simulink model "Expriment_Emotion"  (R2014a)
settings: Solver=FixedStepDiscrete  SolverMode=SingleTasking  StartTime=0.0  StopTime=inf  FixedStep=0.01  RelTol=1e-3
PostLoadFcn:
  | h_RPStest = RPStest;
model workspace (MAT data in the model file):
  gtest = 0
undefined symbols (not defined in the file or in its folder): avert, avert_freq_factor, avert_gaze_dirs_chance, avert_gaze_duration_factor, avert_head_frequency_factor, avert_head_speed, BML, BML1, BML2, bmlsL, bmlsM, bodyBusyFlag, clock, emotion_amount_factor, faceBusyFlag, fileID, GAZE_WIN, gazing, mut_freq_factor, mutual_gaze_duration_factor, P, pose_cat_chance, pose_chanc_factor, pose_chance_factor, pose_frequency_factor, pose_lean, pose_lean_flag, pose_space, pose_speed, pose_twitch, pr, serial, STATE_BEFORE, STATE_GO, STATE_OVER, STATE_READY, Stateflow
libraries: simulink x24, instrumentlib x6, realtime_pacer_lib x2, lib_affectiveChar_behavior x1, lib_affectiveChar_input x1
(part 5 of 6)

== stateflow chart Expriment_Emotion/CharacterControl/personalSpace_Controller ==
  state stateInit
    entry: gameState=14;
    TOO_CLOSE=1;TOO_FAR=2;NEUTRAL=0;
    farBuffer=0;closeBuffer=0;neutralBuffer=0;position=1;
    n=encStr2Arr(' ');bmlsM=[n n n n n];newBmlsM=[n n n n n];
    bmlsL=[n n n n n];newBmlsL=[n n n n n];
  note: Problem:
      | Sometimes locomotion BML is sent (visible in the vhmsgYarpRelais) but it is not running. Also smartbody shows duplicate msg id error. It seems that when too many BMLs are sent to smartbody some of them have same IDs.
  state wait
  note: if avert not 1
  state gazeSurprized
    entry: [P,BMLM]=walkInvadingTable(5) ;
    closeBuffer=closeBuffer+1;
    newBmlsM=insertQueue(bmlsM,BMLM);
    bmlsM=newBmlsM;
  state doIt3Times
    entry: position=2;
    closeBuffer=0;
  note: User is too close!
  state headNeuralGazeCamera
    entry: [P,BMLM]=walkInvadingTable(4) ;
    newBmlsM=insertQueue(bmlsM,BMLM);
    bmlsM=newBmlsM;
  state stateWalkBack
    entry:  [P,BMLM]=walkInvadingTable(2);
    newBmlsM=insertQueue(bmlsM,BMLM);  bmlsM=newBmlsM;
    closeBuffer=closeBuffer+1;
  state browUp
    entry: [P,BMLM]=walkInvadingTable(8) ;
    neutralBuffer=neutralBuffer+1;
    newBmlsM=insertQueue(bmlsM,BMLM);
    bmlsM=newBmlsM;
  state doIt3Times1
    entry: position=1;
    neutralBuffer=0;
  note: EXE ORDER IMPORTANT
  state checkUserCoord
  note: correct: [zChange==1]{position=0;}
  state idle
    entry: [P,BMLM]=walkInvadingTable(1);
    newBmlsM=insertQueue(bmlsM,BMLM);
    bmlsM=newBmlsM;
    neutralBuffer=neutralBuffer+1;
  note: User is in the middle!
  state wait2
  state leanFW
    entry: [P,BMLM]=walkInvadingTable(6) ;
    farBuffer=farBuffer+1;
    newBmlsM=insertQueue(bmlsM,BMLM);
    bmlsM=newBmlsM;
  state doIt3Times2
    entry: position=3;
    farBuffer=0;
  note: Problem:
      | We dont know where smatbody is standing (z pos). If smartbody does not run the locomotion BML sent for any reason (too many BMLs), we want to send locomodation BML again after a while to make sure the personal space is correct. On the other hand, we dont want the module to keep sending move bmls.
  state walkFW
    entry:  [P,BMLM]=walkInvadingTable(3) ;
    newBmlsM=insertQueue(bmlsM,BMLM);  bmlsM=newBmlsM;
    farBuffer=farBuffer+1;
  note: User is too far!
  state leanNeutral
    entry:  [P,BMLM]=walkInvadingTable(7) ;
    newBmlsM=insertQueue(bmlsM,BMLM); bmlsM=newBmlsM;
  (default) -> stateInit
  stateInit -> (junction 2)
  wait -> (junction 2)
  (junction 2) -> headNeuralGazeCamera [order 1] : [avert==1]
  (junction 2) -> checkUserCoord [order 2]
  idle -> wait [order 2] : after(5,secs)
  walkFW -> wait [order 2] : after(5,secs)
  stateWalkBack -> wait [order 2] : after(5,secs)
  doIt3Times1 -> wait : after(5,secs)
  doIt3Times2 -> wait : after(5,secs)
  doIt3Times -> wait : after(5,secs)
  checkUserCoord -> (junction 89) [order 3] : [[distance==TOO_CLOSE]&[position~=2]]
  (junction 89) -> gazeSurprized [order 2] : [closeBuffer<2]
  (junction 89) -> stateWalkBack [order 1] : [closeBuffer>=2]
  stateWalkBack -> doIt3Times [order 1] : [closeBuffer==5]
  gazeSurprized -> checkUserCoord
  headNeuralGazeCamera -> checkUserCoord
  checkUserCoord -> (junction 92) [order 2] : [[distance==NEUTRAL]&[position~=1]]
  (junction 92) -> browUp [order 1] : [neutralBuffer<2]
  wait2 -> checkUserCoord [order 1] : [zChange==1]{position=0;}
  idle -> doIt3Times1 [order 1] : [neutralBuffer==5]
  browUp -> checkUserCoord
  (junction 92) -> idle [order 2] : [neutralBuffer>=2]
  wait2 -> checkUserCoord [order 2] : [zChange~=1]
  checkUserCoord -> wait2 [order 4] : after(20,secs)
  checkUserCoord -> (junction 87) [order 1] : [[distance==TOO_FAR]&[position~=3]]
  leanFW -> checkUserCoord
  (junction 87) -> leanFW [order 2] : [farBuffer<2]
  walkFW -> doIt3Times2 [order 1] : [farBuffer==5]
  (junction 87) -> leanNeutral [order 1] : [farBuffer>=2]
  leanNeutral -> walkFW : after(2,secs)
  data: bmls function_input double size=[1000,5]; myBML function_input double size=[1000,1]; newBmls function_output double size=[1000,5]; p function_output double size=1; bmlID function_input double size=1; poseBML function_output double size=[1000,1]; bmls function_input double size=[1000,5]; myBML function_input double size=[1000,1]; newBmls function_output double size=[1000,5]; gameState output double size=1; STATE_READY data_store_memory size=1; STATE_OVER data_store_memory size=1; distance input double size=1; STATE_BEFORE data_store_memory size=1; BML1 data_store_memory size=[256,1]; P data_store_memory; pr data_store_memory; fileID data_store_memory; neutralBuffer local; closeBuffer local; NEUTRAL local; TOO_FAR local; TOO_CLOSE local; farBuffer local; zChange input; position local; avert data_store_memory; newBmlsM local double size=[1000,5]; bmlsM data_store_memory; BMLM local double size=[1000,1]; BMLL local double size=[1000,1]; newBmlsL local double size=[1000,5]; bmlsL data_store_memory; n local
  events: secs input RISING_EDGE_EVENT
  function newBmls =insertQueueLow(bmls,myBML):
    | function newBmls =insertQueueLow(bmls,myBML)
    |     full=1;
    |     t=encStr2Arr(' ');
    |     newBmls=[t t t t t];
    |     for i = 1:5
    |         if (isequal(bmls(:,i),t))
    |             %add to end of the queue where its empty
    |             bmls(:,i)=myBML;
    |             full=0;
    |             break
    |         end
    |     end
    |     if(full~=0)
    |             %if queue full, shift all elements to left which removes the first one, then add to end
    |             bmls(:,1)= bmls(:,2);
    |             bmls(:,2)= bmls(:,3);
    |             bmls(:,3)= bmls(:,4);
    |             bmls(:,5)=myBML;
    |     end
    |     newBmls=bmls;
  function [p,poseBML]=walkInvadingTable(bmlID):
    | function [p,poseBML]=walkInvadingTable(bmlID)
    | 
    | aVarTruthTableCondition_1 = false;
    | aVarTruthTableCondition_2 = false;
    | aVarTruthTableCondition_3 = false;
    | aVarTruthTableCondition_4 = false;
    | aVarTruthTableCondition_5 = false;
    | aVarTruthTableCondition_6 = false;
    | aVarTruthTableCondition_7 = false;
    | aVarTruthTableCondition_8 = false;
    | 
    | 
    | % n
    | 
    | aVarTruthTableCondition_1 = logical(bmlID==1);
    | 
    | % b
    | 
    | aVarTruthTableCondition_2 = logical(bmlID==2);
    | 
    | % f
    | 
    | aVarTruthTableCondition_3 = logical(bmlID==3);
    | 
    | % HN
    | 
    | aVarTruthTableCondition_4 = logical(bmlID==4);
    | 
    | % surprizeGaze
    | 
    | aVarTruthTableCondition_5 = logical(bmlID==5);
    | 
    | % leanFw
    | 
    | aVarTruthTableCondition_6 = logical(bmlID==6);
    | 
    | % leanNeutral
    | 
    | aVarTruthTableCondition_7 = logical(bmlID==7);
    | 
    | % browUp
    | 
    | aVarTruthTableCondition_8 = logical(bmlID==8);
    | 
    | if (aVarTruthTableCondition_1)
    |     aFcnTruthTableAction_1();
    | elseif (aVarTruthTableCondition_2)
    |     aFcnTruthTableAction_2();
    | elseif (aVarTruthTableCondition_3)
    |     aFcnTruthTableAction_3();
    | elseif (aVarTruthTableCondition_4)
    |     aFcnTruthTableAction_4();
    | elseif (aVarTruthTableCondition_5)
    |     aFcnTruthTableAction_5();
    | elseif (aVarTruthTableCondition_6)
    |     aFcnTruthTableAction_6();
    | elseif (aVarTruthTableCondition_7)
    |     aFcnTruthTableAction_7();
    | elseif (aVarTruthTableCondition_8)
    |     aFcnTruthTableAction_8();
    | else % Default
    |     aFcnTruthTableAction_1();
    | end
    | 
    | function aFcnTruthTableAction_1()
    | 
    | % Neutral
    | 
    | poseBML=encStr2Arr( '<?xml version="1.0" ?><act><bml><locomotion manner="walk" facing="gazeTarget"  sbm:accel="0.5" sbm:scootaccel="50" target="0 0"/></bml></act>');p=1;
    | 
    | function aFcnTruthTableAction_2()
    | 
    | % Back
    | 
    | poseBML=encStr2Arr( '<?xml version="1.0" ?><act><bml><locomotion manner="walk"  sbm:accel="0.5" sbm:scootaccel="50" facing="gazeTarget" target="0 -0.6"/></bml></act>');p=1;
    | 
    | function aFcnTruthTableAction_3()
    | 
    | % Forward
    | 
    | poseBML=encStr2Arr( '<?xml version="1.0" ?><act><bml><locomotion manner="walk" facing="gazeTarget"  sbm:accel="0.5" sbm:scootaccel="50" target="0 0.6"/></bml></act>');p=1;
    | 
    | function aFcnTruthTableAction_4()
    | 
    | % NeutralHead
    | 
    | poseBML=encStr2Arr('<?xml version="1.0" ?><act><bml><gaze target="gazeTarget" sbm:joint-range="EYES NECK" sbm:time-hint="1.5"/></bml></act>');p=1;
    | 
    | function aFcnTruthTableAction_5()
    | 
    | % surprisedGaze
    | 
    | poseBML=encStr2Arr('<?xml version="1.0" ?><act><bml><face type="FACS" start="0" end="5" side="BOTH" au="5" relax="3" amount="0.5"/><face type="FACS" start="0" end="5" side="BOTH" au="2" relax="3" amount="0.5"/></bml></act>');p=1;
    | 
    | function aFcnTruthTableAction_6()
    | 
    | % leanFW
    | 
    | poseBML=encStr2Arr('<?xml version="1.0" ?><act><bml><gaze angle="5" direction="DOWN" sbm:joint-range="HEAD BACK" sbm:time-hint="2" target="gazeTarget"/></bml></act>');p=1;
    | 
    | function aFcnTruthTableAction_7()
    | 
    | % leanNeutral
    | 
    | poseBML=encStr2Arr('<?xml version="1.0" ?><act><bml><gaze sbm:time-hint="2" target="gazeTarget"/></bml></act>');p=1;
    | 
    | function aFcnTruthTableAction_8()
    | 
    | % browUp
    | 
    | poseBML=encStr2Arr('<?xml version="1.0" ?><act><bml><face au="2" end="5" ready="1" relax="4" side="BOTH" start="0" stroke="3" type="facs"/></bml></act>');p=1;
  function newBmls =insertQueue(bmls,myBML):
    | function newBmls =insertQueue(bmls,myBML)
    |     full=1;
    |     t=encStr2Arr(' ');
    |     newBmls=[t t t t t];
    |     for i = 1:5
    |         if (isequal(bmls(:,i),t))
    |             %add to end of the queue where its empty
    |             bmls(:,i)=myBML;
    |             full=0;
    |             break
    |         end
    |     end
    |     if(full~=0)
    |             %if queue full, shift all elements to left which removes the first one, then add to end
    |             bmls(:,1)= bmls(:,2);
    |             bmls(:,2)= bmls(:,3);
    |             bmls(:,3)= bmls(:,4);
    |             bmls(:,5)=myBML;
    |     end
    |     newBmls=bmls;

== stateflow chart Expriment_Emotion/CharacterControl/attention_Controller ==
  state setBodyFlag [parallel]
    settings: executionOrder=1
    state wait
      entry: timer=20;
    state init
      entry: bodyBusyFlag=0;timer=1;
    state flagOne
      entry:  bodyBusyFlag=1;
    state check
    state flagZero
      entry: bodyBusyFlag=0;
    (default) -> init
    init -> check
    flagOne -> wait [order 1] : [body_isAttending==1]
    wait -> flagOne
    check -> flagOne : [body_isAttending==1]
    flagZero -> check
    flagOne -> flagZero [order 2] : after(timer,secs)
  state setFaceFlag [parallel]
    settings: executionOrder=2
    state wait2
      entry: timer2=10;
    state init2
      entry: faceBusyFlag=0;timer2=1;
    state flagOne2
      entry:  faceBusyFlag=1;
    state check2
    state flagZero2
      entry: faceBusyFlag=0;
    (default) -> init2
    init2 -> check2
    flagOne2 -> wait2 [order 1] : [face_isAttending==1]
    wait2 -> flagOne2
    check2 -> flagOne2 : [face_isAttending==1]
    flagZero2 -> check2
    flagOne2 -> flagZero2 [order 2] : after(timer2,secs)
  data: bodyBusyFlag data_store_memory size=1; body_isAttending input; timer local; face_isAttending input; faceBusyFlag data_store_memory size=1; timer2 local
  events: secs input RISING_EDGE_EVENT

== stateflow chart Expriment_Emotion/CharacterControl/facialExpression_Controller ==
  state subSmile [parallel]
    settings: executionOrder=1
    state stateInitial
      entry: avert=1; gameState=14;
      n=encStr2Arr(' ');bmlsM=[n n n n n];newBmlsM=[n n n n n];
    state stateCheckSmile
    state gazeCamera
      entry:  [P,BMLM]= smileTable(2) ;avert=0;
      newBmlsM=insertQueue(bmlsM,BMLM);
      bmlsM=newBmlsM;
    state wait
    state checkP
      entry:  [P,BMLM]=  smileTable(1) ;
      newBmlsM=insertQueue(bmlsM,BMLM);
      bmlsM=newBmlsM;
    (default) -> stateInitial
    stateInitial -> stateCheckSmile : [gameState==20]
    stateCheckSmile -> stateCheckSmile [order 2]
    gazeCamera -> stateCheckSmile [order 2] : after(1,secs)[isSmiling~=1]
    wait -> stateCheckSmile : after(10,secs)
    stateCheckSmile -> gazeCamera [order 1] : [[isSmiling==1]&[ gameState~= STATE_GO]&[ gameState~= STATE_READY]]
    checkP -> wait
    gazeCamera -> checkP [order 1] : after(1,secs)[isSmiling==1]
  note: SMILE_DUER=10 seceonds
  note: check if still isSmiling is true works as a buffer to remove the smiles that last ony 1 sec (system errors).
  state subFacial [parallel]
    settings: executionOrder=2
    state stateFacialExpression
      entry:
      emotion_amount_factor =set_AU_Amount(inA,inV,personality);
      BMLl=cmdBML_AU_VA(emotion_amount_factor);
      newBmlsL=insertQueueLow(bmlsL,BMLl); bmlsL=newBmlsL;
    state initial
    state wait3
    (default) -> initial
    initial -> stateFacialExpression
    wait3 -> stateFacialExpression : after(7,secs)
    stateFacialExpression -> wait3
  data: bmls function_input double size=[1000,5]; myBML function_input double size=[1000,1]; newBmls function_output double size=[1000,5]; bmls function_input double size=[1000,5]; myBML function_input double size=[1000,1]; newBmls function_output double size=[1000,5]; bmlID function_input double; p function_output double size=1; poseBML function_output double size=[1000,1]; bmlID function_input double; p function_output double size=1; poseBML function_output double size=[1000,1]; eAmountFactor function_output double size=[1,11]; arousal function_input double size=1; valence function_input double size=1; inPersonality function_input double size=1; smileN local double size=1; isSmiling input double size=1 =0; avert data_store_memory =0; gazing data_store_memory size=2; GAZE_WIN data_store_memory size=2; BML data_store_memory size=[256,1]; P data_store_memory; fileID local double size=1; gameState output double; STATE_GO data_store_memory; STATE_READY data_store_memory; STATE_BEFORE data_store_memory; newBmlsM local double size=[1000,5]; bmlsM data_store_memory size=[256,1]; BMLM local double size=[1000,1]; n local; personality input double size=1; internalE input double size=1; au local; emotion_amount_factor data_store_memory; aChange input boolean size=1; au_i local double size=1; au_L local double size=1; emoDisp local; bmlsL data_store_memory size=[256,1]; BMLl local double size=[1000,1]; newBmlsL local double size=[1000,5]; emotion_amount_custom input double size=1; inA input double size=1; inV input double size=1; vChange input boolean size=1
  events: secs input RISING_EDGE_EVENT
  function newBmls =insertQueue(bmls,myBML):
    | function newBmls =insertQueue(bmls,myBML)
    |     full=1;
    |     t=encStr2Arr(' ');
    |     newBmls=[t t t t t];
    |     for i = 1:5
    |         if (isequal(bmls(:,i),t))
    |             %add to end of the queue where its empty
    |             bmls(:,i)=myBML;
    |             full=0;
    |             break
    |         end
    |     end
    |     if(full~=0)
    |             %if queue full, shift all elements to left which removes the first one, then add to end
    |             bmls(:,1)= bmls(:,2);
    |             bmls(:,2)= bmls(:,3);
    |             bmls(:,3)= bmls(:,4);
    |             bmls(:,5)=myBML;
    |     end
    |     newBmls=bmls;
  function newBmls =insertQueueLow(bmls,myBML):
    | function newBmls =insertQueueLow(bmls,myBML)
    |     full=1;
    |     t=encStr2Arr(' ');
    |     newBmls=[t t t t t];
    |     for i = 1:5
    |         if (isequal(bmls(:,i),t))
    |             %add to end of the queue where its empty
    |             bmls(:,i)=myBML;
    |             full=0;
    |             break
    |         end
    |     end
    |     if(full~=0)
    |             %if queue full, shift all elements to left which removes the first one, then add to end
    |             bmls(:,1)= bmls(:,2);
    |             bmls(:,2)= bmls(:,3);
    |             bmls(:,3)= bmls(:,4);
    |             bmls(:,5)=myBML;
    |     end
    |     newBmls=bmls;
  function [p,poseBML] = smileTable(bmlID):
    | function [p,poseBML] = smileTable(bmlID)
    | 
    | aVarTruthTableCondition_1 = false;
    | aVarTruthTableCondition_2 = false;
    | 
    | 
    | % smile
    | 
    | aVarTruthTableCondition_1 = logical(bmlID==1);
    | 
    | % headN
    | 
    | aVarTruthTableCondition_2 = logical(bmlID==2);
    | 
    | if (aVarTruthTableCondition_1)
    |     aFcnTruthTableAction_1();
    | elseif (aVarTruthTableCondition_2)
    |     aFcnTruthTableAction_2();
    | else % Default
    |     aFcnTruthTableAction_1();
    | end
    | 
    | function aFcnTruthTableAction_1()
    | 
    | % smile
    | 
    | poseBML=encStr2Arr('<?xml version="1.0"?><act><bml><face amount="1" au="12" side="BOTH" start="0" stroke="2" relax="3" end="4" type="facs"/><face amount="0.3" au="6" side="BOTH" start="0" stroke="2" relax="3" end="4" type="facs"/></bml></act>');p=3;
    | 
    | function aFcnTruthTableAction_2()
    | 
    | % headNeutralBrow
    | 
    | poseBML=encStr2Arr('<?xml version="1.0" ?><act><bml><gaze target="gazeTarget" start="0" end="5" sbm:time-hint="1.5"/></bml></act>');p=3;
    | 
    | function aFcnTruthTableAction_3()
    | 
    | % smileBrow
    | 
    | poseBML=encStr2Arr('<?xml version="1.0"?><act><bml><face amount="0.1" au="1" side="BOTH" start="0" stroke="2" relax="4" end="6" type="facs"/><face amount="0.1" au="2" side="BOTH" start="0" stroke="2" relax="4" end="6" type="facs"/></bml></act>');p=3;
  function [p,poseBML] = facialExpr(bmlID):
    | function [p,poseBML] = facialExpr(bmlID)
    | 
    | aVarTruthTableCondition_1 = false;
    | aVarTruthTableCondition_2 = false;
    | 
    | 
    | % smile
    | 
    | aVarTruthTableCondition_1 = logical(bmlID==1);
    | 
    | % headN
    | 
    | aVarTruthTableCondition_2 = logical(bmlID==2);
    | 
    | if (aVarTruthTableCondition_1)
    |     aFcnTruthTableAction_1();
    | elseif (aVarTruthTableCondition_2)
    |     aFcnTruthTableAction_2();
    | else % Default
    |     aFcnTruthTableAction_1();
    | end
    | 
    | function aFcnTruthTableAction_1()
    | 
    | % smile
    | 
    | poseBML=encStr2Arr('<?xml version="1.0"?><act><bml><face amount="1" au="12" side="BOTH" start="0" stroke="10" relax="70" end="100" type="facs"/><face amount="0.3" au="6" side="BOTH" start="0" stroke="10" relax="70" end="100" type="facs"/></bml></act>');p=3;
    | 
    | function aFcnTruthTableAction_2()
    | 
    | % headNeutralBrow
    | 
    | poseBML=encStr2Arr('<?xml version="1.0" ?><act><bml><gaze target="gazeTarget" start="0" end="5" sbm:time-hint="1.5"/></bml></act>');p=3;
    | 
    | function aFcnTruthTableAction_3()
    | 
    | % smileBrow
    | 
    | poseBML=encStr2Arr('<?xml version="1.0"?><act><bml><face amount="0.1" au="1" side="BOTH" start="0" stroke="2" relax="4" end="6" type="facs"/><face amount="0.1" au="2" side="BOTH" start="0" stroke="2" relax="4" end="6" type="facs"/></bml></act>');p=3;
  function eAmountFactor  =set_AU_Amount(arousal,valence,inPersonality):
    | function eAmountFactor  =set_AU_Amount(arousal,valence,inPersonality)
    | %     15-12-2015, PAD drivern facial expr simul, Grammer data to map AU and VA
    | %     fprintf('VA: %0.0f,%0.0f\r\n',arousal,valence);
    | %     scale
    | %     p = valence * (20/9)  - 10;
    | %     a = arousal * (20/9)  - 10;
    | 
    |     p=valence;a=arousal;
    |     all_AUs=[1,2,4,5,6, 7,12,26,45,10, 25];eAmountFactor=[0,0,0,0,0, 0,0,0,0,0, 0];
    |     for c=1:11
    |         eAmountFactor(1)=0.003*p-0.002*a;  %1,-0.002*a
    |         eAmountFactor(2)=-0.002*p+0.010*a; %2,+0.010*a
    | %         eAmountFactor(12)=-0.016*p+0.034*a; %27 moth open stretch
    |         eAmountFactor(8)=-0.002*p+0.023*a;  %26,-0.002*p+0.049*a
    |         eAmountFactor(5)=-0.008*p+0.009*a;  %6
    |         
    | %         eAmountFactor(13)=0.002*p+0.004*a; %18 lip Puckerer, W 0.3=101
    | %         eAmountFactor(14)=0.007*p+0.025*a; %22 lip fumeler, ShCh 0.5=102       
    | %         eAmountFactor(15)=0.003*p+0.009*a; %14 dimpler FV+PBM 0.5=103
    | %         eAmountFactor(16)=0.003*p+0.009*a; %14 dimpler FV+PBM 0.5=103
    | %         eAmountFactor=-0.010*p+0.017*a;  %17 chin raiser
    | 
    |         eAmountFactor(10)=-0.020*p+0.020*a;  %10 upper lip raiser,-0.053*p+0.026*a
    |         eAmountFactor(4)=-0.003*p+0.032*a; %5 upper lid raiser
    |         eAmountFactor(9)=-0.011*p-0.011*a; %eye closed, 45 instead of 43,-0.021*p-0.037*a
    |         eAmountFactor(3)=-0.036*p+0.022*a; %4 brow lowerer
    | %       eAmountFactor=-0.008*p+0.006*a;    %9 nose wrikler ,10
    | %       eAmountFactor=-0.004*p+0.004*a;    %39?
    | %       eAmountFactor=-0.010*p+0.008*a;    %38?
    | 
    |         eAmountFactor(11)=-0.011*p+0.023*a;%25 lip open,-0.023*p+0.058*a
    | %       eAmountFactor(17)=-0.004*p-0.003*a;    %24 lip pressor, PBM =104       
    | %       eAmountFactor(18)=-0.011*p+0.009*a;    %23 lip tightner PBM0.2 + W0.6=105
    | %       eAmountFactor(19)=-0.011*p+0.009*a;    %23 lip tightner PBM0.2 + W0.6=105
    | 
    | %       eAmountFactor=-0.004*p+0.003*a;    %19?
    | 
    | %       eAmountFactor(20)=0.039*p+0.015*a;  %13 cheek puffer, W 0.3 =106
    |         
    |         eAmountFactor(6)=-0.005*p-0.001*a; %7  Lid Tightener
    |         eAmountFactor(7)=0.057*p+0.009*a;  %12 Lip Corner Puller
    |     %   eAmountFactor=-0.008*p+0.009*a;    %11 Nasolabial Deepener
    |     %   eAmountFactor=-0.046*p-0.002*a;    %15 Lip Corner Depressor
    |     %   eAmountFactor=-0.014*p+0.016*a;    %16 Lower Lip Depressor
    |     %   eAmountFactor(20)=-0.026*p+0.010*a;%20 lip stretch
    |         
    |         eAmountFactor=eAmountFactor/6; %scale
    |         if(inPersonality==2 || inPersonality==4)%introvert
    |             eAmountFactor=eAmountFactor/1.3; % divide by 4/3
    |         end
    |     end

== matlab function Expriment_Emotion/EmotionSubsystem/calculateValenceArousal/LEHN_VA_Emo ==
  data: V input; e output double size=1; A input double
function e = fcn(V, A)

aVarTruthTableCondition_1 = false;
aVarTruthTableCondition_2 = false;
aVarTruthTableCondition_3 = false;
aVarTruthTableCondition_4 = false;
aVarTruthTableCondition_5 = false;
aVarTruthTableCondition_6 = false;
aVarTruthTableCondition_7 = false;
aVarTruthTableCondition_8 = false;


% 7-happy  2,1

aVarTruthTableCondition_1 = logical(V>20 && A<40 && A>20);

% 8-ex  1,2 AND 2,2

aVarTruthTableCondition_2 = logical(V>0 && A>40);

% 4-fear  -1,2 AND -2,2

aVarTruthTableCondition_3 = logical(V<0 && A>40);

% 3-frust  -2,1

aVarTruthTableCondition_4 = logical(V<-20 && A<40 && A>20);

% 6-idle  2,-1

aVarTruthTableCondition_5 = logical(V>20 && A<-20 && A>-40);

% 5-calm  1,-2 AND 2,-2

aVarTruthTableCondition_6 = logical(V>0 && A<-40);

% 1-bored  -1,-2 AND -2,-2

aVarTruthTableCondition_7 = logical(V<0 && A<-40);

% 2-sad  -2,-1

aVarTruthTableCondition_8 = logical(V<-20 && A<-20 && A>-40);

if (aVarTruthTableCondition_1)
    aFcnTruthTableAction_1();
elseif (aVarTruthTableCondition_2)
    aFcnTruthTableAction_2();
elseif (aVarTruthTableCondition_3)
    aFcnTruthTableAction_3();
elseif (aVarTruthTableCondition_4)
    aFcnTruthTableAction_4();
elseif (aVarTruthTableCondition_5)
    aFcnTruthTableAction_5();
elseif (aVarTruthTableCondition_6)
    aFcnTruthTableAction_6();
elseif (aVarTruthTableCondition_7)
    aFcnTruthTableAction_7();
elseif (aVarTruthTableCondition_8)
    aFcnTruthTableAction_8();
else % Default
    aFcnTruthTableAction_5();
end

function aFcnTruthTableAction_1()

% happy

e=7;

function aFcnTruthTableAction_2()

% excited

e=8;

function aFcnTruthTableAction_3()

% fear

e=4;

function aFcnTruthTableAction_4()

% frustration

e=3;

function aFcnTruthTableAction_5()

% idle

e=6;

function aFcnTruthTableAction_6()

% contempt

e=5;

function aFcnTruthTableAction_7()

% bored

e=1;

function aFcnTruthTableAction_8()

% sad

e=2;

== matlab function Expriment_Emotion/EmotionSubsystem/satFunction ==
  data: randv input; smile input; wave input; win input; invade input; v_trigW output; vaFlag input; v_trig output
function [v_trigW,v_trig]= fcn(randv,smile,wave,win,invade,vaFlag)
%#codegen
% 30/06/2015
    %Here set Agent's satisfaction flag based on your scenario
    %In RPS scenario agent gets satisfined when she wins. states of interaction= {STATE_READY=7;
    %STATE_GO=1;STATE_HAND=2;STATE_OVER=3; STATE_BEFORE=4;STATE_RESULT=5;STATE_WAIT=6;}
   
    if(vaFlag==1)
        v_trigW=0;%weight by which valence value is changed (sum of weight of all triggers)
        %randv 30% chance of random increase or decrease in valence
        randTrigger=floor(randv);
        if(0<randTrigger)&&(randTrigger<30)
            v_trigW = v_trigW + 0.6;
        end
        if(30<randTrigger)&&(randTrigger<60)
            v_trigW = v_trigW - 0.6;
        end

        if(win==2) %agent wins so she is satisfied
            v_trigW = v_trigW + 0.5;
        elseif(win==1) %user wins so agent is NOT satisfied
            v_trigW = v_trigW - 0.5;
        end

        if(smile==1)
            v_trigW=v_trigW+0.25;
        end

        if(wave==1)
            v_trigW=v_trigW+0.25;
        end

        if(invade==1)
            v_trigW=v_trigW-0.25;
        end
    else
         v_trigW=0;
    end
    if(v_trigW>0)
        v_trig=1;
    elseif(v_trigW<0)
        v_trig=-1;
        v_trigW=abs(v_trigW);
    else
        v_trig=0;
    end

== matlab function Expriment_Emotion/EmotionSubsystem/arousalFlagFunction ==
  data: userInvade input; interactionState input; a_trig output; a_trigW output; vaFlag input; randa input
function [a_trig,a_trigW]= fcn(userInvade,interactionState,vaFlag,randa)
%#codegen
% 30/06/2015
    %Here set in which states of the interaction agent experienced 
    % more arousal(arousalFlag=1) and less arousal (arousalFlag=-1)
    %Note that you should define the states in your scenraio beforehand
    %we assume agent gets more aroused when in ready/go state and 
    %less aroused when in WAITE/HAND
    if(vaFlag==1)
        a_trigW=0; %weight by which arousal value is changed (sum of weight of all triggers)

        %randa 30% chance of random increase or decrease in arousal
        randTrigger=floor(randa);
        if(0<randTrigger)&&(randTrigger<30)
            a_trigW=a_trigW + 0.6;
        end
        if(30<randTrigger)&&(randTrigger<60)
            a_trigW=a_trigW - 0.6;
        end

        if(interactionState==1)%GO - highely aroused state
            a_trigW=a_trigW+0.5;
        end
        if(interactionState==7)%READY - high aroused state
            a_trigW=a_trigW+0.5;
        end
        if(interactionState==2)%HAND- highely aroused state
            a_trigW=a_trigW -0.5;
        end
        if(interactionState==6)%WAIT - low aroused state
            a_trigW=a_trigW-0.5;
        end
        %     elseif(interactionState==3)%OVER - low aroused state
    %         arousalTrig=-1;  
    %         end
        if(userInvade==1)
           a_trigW=a_trigW+0.25;
        end
    else
        a_trigW=0;
    end
    if(a_trigW>0)
        a_trig=1;
    elseif(a_trigW<0)
        a_trig=-1;
        a_trigW=abs(a_trigW);
    else
        a_trig=0;
    end

== stateflow chart Expriment_Emotion/GazeFollowSubsystem/reactiveGaze/createGazePawn ==
  state sendBML(In1) [function]
  state sendSBM(In2) [function]
  state stateCreatePawn
    entry:
    sendSBM( encStr2Arr( 'gt = scene.createPawn("gazeTarget")' ) );
    sendBML(encStr2Arr('<?xml version="1.0" ?><act><bml><gaze sbm:joint-range="EYES BACK" target="gazeTarget"/></bml></act>'));
  (default) -> stateCreatePawn
  data: In1 function_input double size=[1000 1]; In2 function_input double size=[1000 1]

== matlab function Expriment_Emotion/GazeFollowSubsystem/reactiveGaze/reactiveGazeControl/reactiveMovePawn ==
  data: x input; y input; arrBML output
function arrBML   = fcn( x,y )
    coder.extrinsic('sprintf')
    %for agent to gaze at the user, we create a pawn where user stands and agent gazes at the pawn
    %1) AnTS: x btw 200,600/gaze btw -0.3,0.3
    %2) Kinect: x btw -80,80/gaze btw -0.2,0.2
    %3) newKinect: x btw -100,100/gaze btw -0.2,0.2
    %changed from x,1.8,2.5 to x,3,10

    %x=(x-200)/600;
    %x=x/400; %80/0.2
    x=x/500; %100/0.2
    c = countDigits(x);
    mystr=blanks(77+c);
    %mystr = sprintf('scene.getPawn(\"gazeTarget\").setPosition(SrVec(%d, %d ,%d))',x,0,150);
    mystr = sprintf('scene.getPawn(\"gazeTarget\").setPosition(SrVec(%0.3f , %0.1f ,%0.1f))',x,1.6,10); %x btw 0,1

    arrBML = encStr2Arr(mystr);
end

== matlab function Expriment_Emotion/randomArray/makleArray ==
  data: r1 input; y output double size=[1,40]; r2 input; r3 input; r4 input; r5 input; r6 input; r7 input; r8 input; r9 input; r10 input; r11 input; r12 input; r13 input; r14 input; r15 input; r16 input; r17 input; r18 input; r19 input; r20 input; r21 input; r22 input; r23 input; r24 input; r25 input; r26 input; r27 input; r28 input; r29 input; r30 input; r31 input; r32 input; r33 input; r34 input; r35 input; r36 input; r37 input; r38 input; r39 input; r40 input
function y = fcn(r1,r2,r3,r4,r5,r6,r7,r8,r9,r10,r11,r12,r13,r14,r15,r16, r17, r18, r19,r20,r21,r22,r23,r24,r25,r26,r27,r28,r29,r30,r31,r32,r33,r34,r35,r36,r37,r38,r39,r40)
%#codegen
y=[0,0,0,0,0,0,0,0,0,0,  0,0,0,0,0,0,0,0,0,0,  0,0,0,0,0,0,0,0,0,0,  0,0,0,0,0,0,0,0,0,0];
y(:,1) = floor(r1);
y(:,2) = floor(r2);
y(:,3) = floor(r3);
y(:,4) = floor(r4);
y(:,5) = floor(r5);
y(:,6) = floor(r6);
y(:,7) = floor(r7);
y(:,8) = floor(r8);
y(:,9) = floor(r9);
y(:,10) = floor(r10);
y(:,11) = floor(r11);
y(:,12) = floor(r12);
y(:,13) = floor(r13);
y(:,14) = floor(r14);
y(:,15) = floor(r15);
y(:,16) = floor(r16);
y(:,17) = floor(r17);
y(:,18) = floor(r18);
y(:,19) = floor(r19);
y(:,20) = floor(r20);
y(:,21) = floor(r21);
y(:,22) = floor(r22);
y(:,23) = floor(r23);
y(:,24) = floor(r24);
y(:,25) = floor(r25);
y(:,26) = floor(r26);
y(:,27) = floor(r27);
y(:,28) = floor(r28);
y(:,29) = floor(r29);
y(:,30) = floor(r30);
y(:,31) = floor(r31);
y(:,32) = floor(r32);
y(:,33) = floor(r33);
y(:,34) = floor(r34);
y(:,35) = floor(r35);
y(:,36) = floor(r36);
y(:,37) = floor(r37);
y(:,38) = floor(r37);
y(:,39) = floor(r39);
y(:,40) = floor(r40);

== matlab function Expriment_Emotion/facialExpr/checkNeutral ==
  data: notNeutral output double size=1; e input
function notNeutral = fcn(e)
%#codegen

if(e~=6)
    notNeutral=1;
else
    notNeutral=0;
end

== matlab function Expriment_Emotion/GazeFollowSubsystem/gazeFollow ==
  data: state input; stateOver output
function stateOver = fcn(state)
%#codegen

%Maryam 30/06/2015
%Here set in which states of the interaction agent experienced 
% more arousal(arousalFlag=1) and less arousal (arousalFlag=-1)

%Note that you should define the states in your scenraio beforehand

%we assume agent gets more aroused when in ready/go state and 
%less aroused when in WAITE/HAND

if(state==3)%only gaze follows user in ganme-over states 
                      %since in other states we assume user is not moving
    stateOver=1;
else
    stateOver=0;

end

== stateflow chart Expriment_Emotion/CharacterControl/wave_Controller ==
  state init
    entry: STATE_OVER=3;
    STATE_BEFORE=4;
    gameState=14;
    rFlag=0;lFlag=0;bFlag=0;
    n=encStr2Arr(' ');bmlsM=[n n n n n];
    newBmlsM=[n n n n n];
  state waveRightHand
    entry: [P,BMLM]= wavePoseBradTable(1+animNum);
    rFlag=1;
    newBmlsM=insertQueue(bmlsM,BMLM);
    bmlsM=newBmlsM;
  state gazeCamera
    entry: [P,BMLM]= wavePoseBradTable(8);
    avert=0;
    newBmlsM=insertQueue(bmlsM,BMLM);
    bmlsM=newBmlsM;
  state wave
    entry: animNum =setPersonalityParams(personality);
  state waveLeftHand
    entry:
    [P,BMLM]= wavePoseBradTable(animNum);
    lFlag=1;
    newBmlsM=insertQueue(bmlsM,BMLM);
    bmlsM=newBmlsM;
  state gazeCamera1
    entry: [P,BMLM]= wavePoseBradTable(8);
    avert=0;
    newBmlsM=insertQueue(bmlsM,BMLM);
    bmlsM=newBmlsM;
  note: if introvert 50% chance of introvertWave(poseN=7)
  note: else(extrovert)
  state gazeCamera2
    entry: [P,BMLM]= wavePoseBradTable(8);
    avert=0;
    newBmlsM=insertQueue(bmlsM,BMLM);
    bmlsM=newBmlsM;
  state waveBothHands
    entry: [P,BMLM]= wavePoseBradTable(3+animNum);
    bFlag=1;
    newBmlsM=insertQueue(bmlsM,BMLM);
    bmlsM=newBmlsM;
  note: Problem with procedural behaviors (you can not give duration and they stay in that pose untill new bml comes so they dont return to idle)
      | we want the agent to gaze at user for the period of waving.If new idle gaze BML comes, agent averts gaze or head before wave finished. Gaze is procedural (gazes at the point till new gaze bml is recieved so it does not automatically return to idle pose) so we can not give duration of gaze in the BML. The only way to avoid avert during wave is to make sure thre is no idle gaze bmls during the wave; which makes sense considering the gaze does not avert(idle) when you are attending something.
      | prioritizing does not solve this because avertGaze comes right after gazeCamera and wave. We also can not delay after high priorities because sometime several high priorities should happen right after eachother.
  waveBothHands -> wave : after(5,secs)
  waveRightHand -> wave : after(5,secs)
  waveLeftHand -> wave : after(5,secs)
  (default) -> init
  init -> wave
  (junction 55) -> waveRightHand [order 2]
  gazeCamera -> waveRightHand : after(2,secs)
  wave -> (junction 55) [order 4] : [[handUp==1]&[rFlag==0]]{ lFlag=0;bFlag=0;}
  (junction 55) -> gazeCamera [order 1] : [avert==1]
  wave -> wave [order 1] : after(10,secs){ rFlag=0;lFlag=0;bFlag=0;}
  wave -> (junction 59) [order 3] : [[handUp==3]&[bFlag==0]]{ rFlag=0;lFlag=0;}
  wave -> (junction 58) [order 2] : [[handUp==2]&[lFlag==0]]{ rFlag=0;bFlag=0;}
  (junction 82) -> waveLeftHand [order 1] : [randP==1]{animNum=7;}
  (junction 58) -> (junction 79) [order 2]
  (junction 79) -> (junction 82) [order 1] : [[personality==2]|[personality==4]]{randP=randArray(:,12)}
  (junction 58) -> gazeCamera1 [order 1] : [avert==1]
  gazeCamera1 -> (junction 79) : after(2,secs)
  (junction 79) -> waveLeftHand [order 2] : {animNum=2+animNum;}
  (junction 82) -> waveLeftHand [order 2] : [randP==2]{animNum=2+animNum;}
  (junction 59) -> waveBothHands [order 2]
  (junction 59) -> gazeCamera2 [order 1] : [avert==1]
  gazeCamera2 -> waveBothHands : after(2,secs)
  data: pr function_output double size=1; bmlID function_input double; poseBML function_output double size=[1000,1]; num function_output double size=1; p function_input double size=1; bmls function_input double size=[1000,5]; mBML function_input double size=[1000,1]; newBmls function_output double size=[1000,5]; fileID data_store_memory; handUp input; gameState output double size=1; BML data_store_memory; P data_store_memory; STATE_OVER data_store_memory; STATE_BEFORE data_store_memory; rFlag local; lFlag local; bFlag local; BML2 data_store_memory; avert data_store_memory; BMLM local double size=[1000,1]; newBmlsM local double size=[1000,5]; bmlsM data_store_memory; n local; personality input double size=1; randP local; animNum local; randArray input double size=[1,40]; personalityChange input boolean size=1
  events: secs input RISING_EDGE_EVENT
  function [pr,poseBML]=wavePoseBradTable(bmlID):
    | function [pr,poseBML]=wavePoseBradTable(bmlID)
    | 
    | aVarTruthTableCondition_1 = false;
    | aVarTruthTableCondition_2 = false;
    | aVarTruthTableCondition_3 = false;
    | aVarTruthTableCondition_4 = false;
    | aVarTruthTableCondition_5 = false;
    | aVarTruthTableCondition_6 = false;
    | aVarTruthTableCondition_7 = false;
    | aVarTruthTableCondition_8 = false;
    | aVarTruthTableCondition_9 = false;
    | aVarTruthTableCondition_10 = false;
    | 
    | 
    | 
    | aVarTruthTableCondition_1 = logical(bmlID==1);
    | 
    | 
    | aVarTruthTableCondition_2 = logical(bmlID==2);
    | 
    | 
    | aVarTruthTableCondition_3 = logical(bmlID==3);
    | 
    | 
    | aVarTruthTableCondition_4 = logical(bmlID==4);
    | 
    | 
    | aVarTruthTableCondition_5 = logical(bmlID==5);
    | 
    | 
    | aVarTruthTableCondition_6 = logical(bmlID==6);
    | 
    | 
    | aVarTruthTableCondition_7 = logical(bmlID==7);
    | 
    | 
    | aVarTruthTableCondition_8 = logical(bmlID==8);
    | 
    | 
    | aVarTruthTableCondition_9 = logical(bmlID==9);
    | 
    | 
    | aVarTruthTableCondition_10 = logical(bmlID==10);
    | 
    | if (aVarTruthTableCondition_1)
    |     aFcnTruthTableAction_1();
    | elseif (aVarTruthTableCondition_2)
    |     aFcnTruthTableAction_2();
    | elseif (aVarTruthTableCondition_3)
    |     aFcnTruthTableAction_3();
    | elseif (aVarTruthTableCondition_4)
    |     aFcnTruthTableAction_4();
    | elseif (aVarTruthTableCondition_5)
    |     aFcnTruthTableAction_5();
    | elseif (aVarTruthTableCondition_6)
    |     aFcnTruthTableAction_6();
    | elseif (aVarTruthTableCondition_7)
    |     aFcnTruthTableAction_7();
    | elseif (aVarTruthTableCondition_8)
    |     aFcnTruthTableAction_8();
    | elseif (aVarTruthTableCondition_9)
    |     aFcnTruthTableAction_9();
    | elseif (aVarTruthTableCondition_10)
    |     aFcnTruthTableAction_10();
    | else % Default
    |     aFcnTruthTableAction_1();
    | end
    | 
    | function aFcnTruthTableAction_1()
    | 
    | % waveLeftF
    | 
    | poseBML=encStr2Arr('<?xml version="1.0" ?><act><bml><animation name="../data/ChrBrad/test_wave_left.skm" speed="2"/></bml></act>'); pr=2;
    | 
    | function aFcnTruthTableAction_2()
    | 
    | % waveRightF
    | 
    | poseBML=encStr2Arr('<?xml version="1.0" ?><act><bml><animation name="../data/ChrBrad/test_wave_right.skm" speed="2"/></bml></act>'); pr=2;
    | 
    | function aFcnTruthTableAction_3()
    | 
    | % waveBothF
    | 
    | poseBML=encStr2Arr('<?xml version="1.0" ?><act><bml><animation name="ChrBrad@Idle01_BeatHighBt01" speed="2"/></bml></act>'); pr=2;
    | 
    | function aFcnTruthTableAction_4()
    | 
    | % waveLeftSlow
    | 
    | poseBML=encStr2Arr('<?xml version="1.0" ?><act><bml><animation name="../data/ChrBrad/test_wave_left.skm" speed="0.5"/></bml></act>'); pr=2;
    | 
    | function aFcnTruthTableAction_5()
    | 
    | % WaveRightSlow
    | 
    | poseBML=encStr2Arr('<?xml version="1.0" ?><act><bml><animation name="../data/ChrBrad/test_wave_right.skm" speed="0.5"/></bml></act>'); pr=2;
    | 
    | function aFcnTruthTableAction_6()
    | 
    | % WaveBothSlow
    | 
    | poseBML=encStr2Arr('<?xml version="1.0" ?><act><bml><animation name="ChrBrad@Idle01_BeatHighBt01" speed="0.5"/></bml></act>'); pr=2;
    | 
    | function aFcnTruthTableAction_7()
    | 
    | % WaveLIntrovert
    | 
    | poseBML=encStr2Arr('<?xml version="1.0" ?><act><bml><animation name="../data/ChrBrad/test_introvert_wave.skm" speed="1"/></bml></act>'); pr=2;
    | 
    | function aFcnTruthTableAction_8()
    | 
    | % gazeCamera
    | 
    | poseBML=encStr2Arr('<?xml version="1.0" ?><act><bml><gaze target="gazeTarget" sbm:joint-range="EYES NECK" sbm:time-hint="1.5"/></bml></act>');pr=2;
    | 
    | function aFcnTruthTableAction_9()
    | 
    | % waveLeft
    | 
    | poseBML=encStr2Arr('<?xml version="1.0" ?><act><bml><animation name="ChrBrad@Idle01_BeatHighRt01"/></bml></act>');pr=2;
    | 
    | function aFcnTruthTableAction_10()
    | 
    | % waveRight
    | 
    | poseBML=encStr2Arr('<?xml version="1.0" ?><act><bml><animation name="ChrBrad@Idle01_BeatHighRt01"/></bml></act>');pr=2;
  function num =setPersonalityParams(p):
    | function num =setPersonalityParams(p)
    |  num=0;
    |  if(p==1) %HE
    |     num=0;
    |  elseif(p==2)%LE
    |     num=3;
    |  elseif(p==3)%HE
    |     num=0;
    |  else%LE
    |     num=3;
    |  end
  function newBmls =insertQueue(bmls,mBML):
    | function newBmls =insertQueue(bmls,mBML)
    |     full=1;
    |     t=encStr2Arr(' ');
    |     newBmls=[t t t t t];
    |     for i = 1:5
    |         if (isequal(bmls(:,i),t))
    |             %add to end of the queue where its empty
    |             bmls(:,i)=mBML;
    |             full=0;
    |             break
    |         end
    |     end
    |     if(full~=0)
    |             %if queue full, shift all elements to left which removes the first one, then add to end
    |                         disp('before add when full');disp(bmls);
    |             bmls(:,1)= bmls(:,2);
    |             bmls(:,2)= bmls(:,3);
    |             bmls(:,3)= bmls(:,4);
    |             bmls(:,5)=mBML;
    |             
    |     end
    |     newBmls=bmls;

== matlab function Expriment_Emotion/handUpTable ==
  data: R input; L input; y output
function y = fcn(R, L)

aVarTruthTableCondition_1 = false;
aVarTruthTableCondition_2 = false;
aVarTruthTableCondition_3 = false;
aVarTruthTableCondition_4 = false;


% no hand up

aVarTruthTableCondition_1 = logical(R==0 && L==0);

% right hand up

aVarTruthTableCondition_2 = logical(R==1 && L==0);

% left hand up

aVarTruthTableCondition_3 = logical(R==0 && L==1);

% both hands up

aVarTruthTableCondition_4 = logical(R==1 && L==1);

if (aVarTruthTableCondition_1)
    aFcnTruthTableAction_1();
elseif (aVarTruthTableCondition_2)
    aFcnTruthTableAction_2();
elseif (aVarTruthTableCondition_3)
    aFcnTruthTableAction_3();
elseif (aVarTruthTableCondition_4)
    aFcnTruthTableAction_4();
else % Default
    aFcnTruthTableAction_1();
end

function aFcnTruthTableAction_1()

% no hand up

y = 0;

function aFcnTruthTableAction_2()

% right hand up

y = 1;

function aFcnTruthTableAction_3()

% left hand up

y = 2;

function aFcnTruthTableAction_4()

% both hands up

y = 3;

== matlab function Expriment_Emotion/facialExpr/facialExprGen/setAU ==
  data: E input double size=1; AU output double size=[1,6]; L output double size=1
function [AU,L]=setAU(E)	
% 1	Inner Brow Raiser,% 2	Outer Brow Raiser, % 4	Brow Lowerer
% 5	Upper Lid Raiser,% 6	Cheek Raiser,% 7	Lid Tightener
% 8	Lips Toward Each Other,% 9	Nose Wrinkler,% 10	Upper Lip Raiser	
% 11	Nasolabial Deepener	% 12	Lip Corner Puller % 13	Sharp Lip Puller % 14	Dimpler	
% 15	Lip Corner Depressor % 16	Lower Lip Depressor % 17	Chin Raiser	mentalis
% 18	Lip Pucker	% 19	Tongue Show	% 20	Lip Stretcher % 21	Neck Tightener	platysma
% 22	Lip Funneler% 23	Lip Tightener% 24	Lip Pressor % 25	Lips Part	depressor
% 26	Jaw Drop,% 27	Mouth Stretch
% 43	Eyes Closed, % 44	Eyebrow Gatherer,% 45	Blink,% 46	Wink
%smartbody no 43,15,17,10 looks wierd,no 142
   AU=[6,12,142,0,0,0];L=3;
   % AU5(eyeOpen) for A+
   % AU1,4 for V-
   %AU12 for V+
    switch(E)
        case 1 %V- A-,bored (43)[1]
            AU=[1,2,45,0,0,0];L=3;%[1,1,0.35]
        
        case 2 %V- A-;sad %(1,2,4,10,15,17,43)[];can be [1,2,4,45,6,0]
            AU=[1,4,0,0,0,0];L=2;%[1,1,0,0,0,0]
        
        case 3 %V- A+,frust(2,1,14)[1],(-1,-2,4,7,14)[2], maybe(1,7)[0.7,0.7,0.5]
            AU=[1,2,4,5,6,0];L=5;%[1,1,1,0.5,0.5,0]
        
        case 4 %V- A+,fear(1,2,4,5,25=mouth)
            AU=[1,2,4,5,6,7];L=6; %[1,1,1,0.2,0.2]
        
        case 5%V+ A-,calm,sleepy
            AU=[12,14,0,0,0,0];L=2;%[0.7,0.3,0,0,0,0]
        
        case 7%V+ A+,happy
            AU=[6,12,0,0,0,0];L=2;%[1,0.5,0,0,0,0]
        
        case 8%V+ A+,excited
            AU=[12,26,5,1,2,0];L=5;%[1,1,1,1,1,0]
        
        case 9%V- A+, angry
            AU=[2,4,5,7,45,0];L=5;%[0.5,1,0.2,0.2,0.2]
        
        otherwise
            %confusion (1,2,4,7)[1] %[1,1,1,0.2]
            %worried (1,2,4,5) [1,1,1,0.5]
            %angry(4,5,7,10,27)[], can be(2,4,5,7,45)[0.5,1,0.2,0.2,0.2]

            AU=[4,7,12,0,0,0];L=3;
            disp('error, emotion not listed:');disp(E);
    end  
%[1]Craig S.D. et al(2004)emotions during learning:the first steps tw affect sensitive
%[2]grafsgard J F () automatically recog facial indicator of frust

== matlab function Expriment_Emotion/facialExpr/facialExprGen/forloop/displayBMLs ==
  data: e input; l input; i input double size=1 [1..]; bml input
function fcn(e,l,i,bml)
%#codegen
fprintf('%s','e:');fprintf('%f',e);
fprintf('%s','  ,L:');fprintf('%f',l);
fprintf('%s','  ,i:');fprintf('%f',i);
disp(decArr2Str(bml));

== matlab function Expriment_Emotion/readSHORE/smile/ifSmile ==
  data: u input; y output
function y = fcn(u)
%#codegen
if u>0.5
    smile=1;
else
    smile=0;
end
y = smile;

== matlab function Expriment_Emotion/facialExpr/facialExprGen/setAmount ==
  data: E input double size=1; eAmountFactor output double size=[1,6]; Pt input double size=1
function eAmountFactor =setAmount(E,Pt)
    AU=[6,12,142,0,0,0];eAmountFactor=[1,1,1,0,0,0];pFactor=1;
    
    if(Pt==1)
        %HEHN
        if(E==1)  %bored
            eAmountFactor=[1,1,0,0.35,0,0];
        elseif(E==2) %sad
            eAmountFactor=[1,1,0,0,0,0];
        elseif(E==3) %frust
            eAmountFactor=[1,1,1,0.5,0.5,0];
        elseif(E==4) %fear
            eAmountFactor=[1,1,1,0.2,0.2,0];
        elseif(E==5)%sleepy
            eAmountFactor=[0.7,0.3,0.3,0,0,0];
        elseif(E==7)%happy
            eAmountFactor=[1,0.5,0,0,0,0];
        elseif(E==8)%excited
            eAmountFactor=[1,1,1,1,1,0];    
        else          
            eAmountFactor=[1,1,1,0,0,0];
            disp('error, emotion not listed:');disp(E);
        end
    
        %LEHN  
    elseif(Pt==2)
       if(E==1)  %bored
            eAmountFactor=[1,1,0,0.35,0,0];
        elseif(E==2) %sad
            eAmountFactor=[1,1,0,0,0,0];
        elseif(E==3) %frust
            eAmountFactor=[1,1,1,0.5,0.5,0];
        elseif(E==4) %fear
            eAmountFactor=[1,1,1,0.2,0.2,0];
        elseif(E==5)%sleepy
            eAmountFactor=[0.7,0.3,0.3,0,0,0];
        elseif(E==7)%happy
            eAmountFactor=[1,0.5,0,0,0,0];
        elseif(E==8)%excited
            eAmountFactor=[1,1,1,1,1,0];    
        else          
            eAmountFactor=[1,1,1,0,0,0];
            disp('error, emotion not listed:');disp(E);
        end

        %HELN
   elseif(Pt==3)
        if(E==1)  %bored
            eAmountFactor=[1,1,0,0.35,0,0];
        elseif(E==2) %sad
            eAmountFactor=[1,1,0,0,0,0];
        elseif(E==3) %frust
            eAmountFactor=[1,1,1,0.5,0.5,0];
        elseif(E==4) %fear
            eAmountFactor=[1,1,1,0.2,0.2,0];
        elseif(E==5)%sleepy
            eAmountFactor=[0.7,0.3,0.3,0,0,0];
        elseif(E==7)%happy
            eAmountFactor=[1,0.5,0,0,0,0];
        elseif(E==8)%excited
            eAmountFactor=[1,1,1,1,1,0];    
        else          
            eAmountFactor=[1,1,1,0,0,0];
            disp('error, emotion not listed:');disp(E);
        end
        eAmountFactor=eAmountFactor*pFactor;
        %LELN
    elseif(Pt==4)
        if(E==1)  %bored
            eAmountFactor=[1,1,0,0.35,0,0];
        elseif(E==2) %sad
            eAmountFactor=[1,1,0,0,0,0];
        elseif(E==3) %frust
            eAmountFactor=[1,1,1,0.5,0.5,0];
        elseif(E==4) %fear
            eAmountFactor=[1,1,1,0.2,0.2,0];
        elseif(E==5)%sleepy
            eAmountFactor=[0.7,0.3,0.3,0,0,0];
        elseif(E==7)%happy
            eAmountFactor=[1,0.5,0,0,0,0];
        elseif(E==8)%excited
            eAmountFactor=[1,1,1,1,1,0];    
        else          
            eAmountFactor=[1,1,1,0,0,0];
            disp('error, emotion not listed:');disp(E);
        end
        eAmountFactor=eAmountFactor*pFactor;
    end
%Following is if we want a same factor for each personaliy all through AUs
% function eAmountFactor =set_eAmountFactor(E,P)
%     AU=[6,12,142,0,0,0];eAMOUNT=[0,0,0,0,0,0];
%     switch E
%         case 1  %bored
%             eAMOUNT=[1,1,1,0,0,0];
%         case 2 %sad
%             eAMOUNT=[0.7,0.4,0.9,0,0,0];
%         case 3 %angry
%             eAMOUNT=[1,0.8,1,0,0,0];
%         case 4 %fear
%             eAMOUNT=[1,1,1,0,0,0];%5,6,7,26
%         case 5%contempt
%             eAMOUNT=[1,1,1,0,0,0];
%         case 7%happy
%             eAMOUNT=[0.2,1,0,0,0,0];
%         otherwise           
%             eAMOUNT=[0,0,0,0,0,0];
%             disp('error,amount for emotion not listed:');disp('eAMOUNT');
%     end 
%     switch P
%         case 1 %HEHN
%             pFactor=1;
%         case 2 %LEHN
%             pFactor=1;
%         case 3 %HELN
%             pFactor=0.5;
%         case 4 %LELN
%             pFactor=0.5;
%     end
%     eAmountFactor=pFactor*eAMOUNT;

== matlab function Expriment_Emotion/facialExpr/facialExprGen/emotionBMLsLoop/displayBMLs ==
  data: e input; i input double size=1 [1..]; bml input
function fcn(e,i,bml)
%#codegen
fprintf('%f',e);
fprintf('%d',i);
disp(decArr2Str(bml));
